simulink model "Milestone1"  (R2022b)
settings: Solver=VariableStepAuto  StartTime=0.0  StopTime=32  RelTol=1e-3
libraries: simulink x5
settings Model: Creator=nhatbuiminh  LastModifiedBy=nhatbuiminh

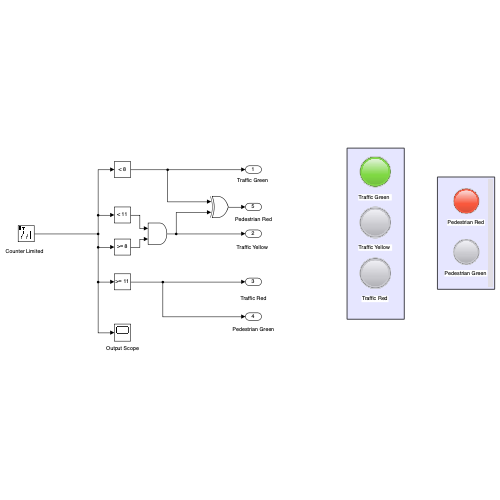
[thumbnail: Simulink's stored preview of the top-level diagram]
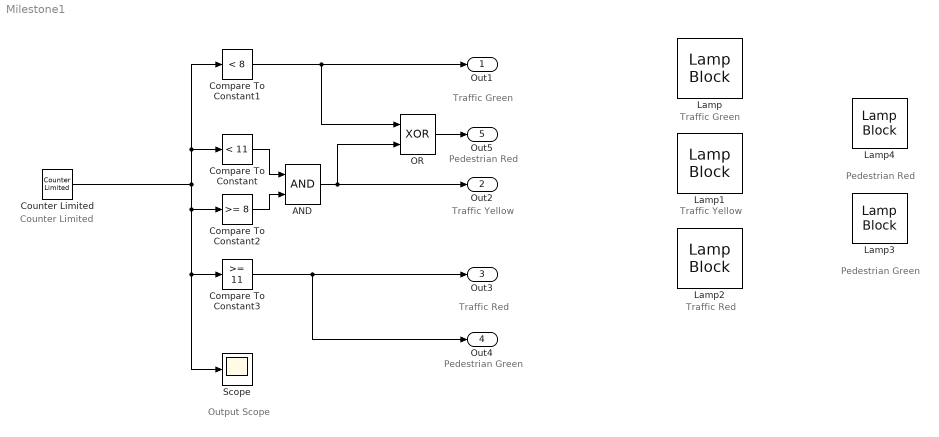
== system Milestone1 ==
  note: Pedestrian Green
  note: Traffic Red
  note: Traffic Yellow
  note: Traffic Green
  note: Traffic Green
  note: Traffic Yellow
  note: Traffic Red
  note: Pedestrian Green
  note: Pedestrian Red
  note: Pedestrian Red
  note: Output Scope
  note: Counter Limited
  AND : Logic  IconShape=distinctive  AllPortsSameDT=off  OutDataTypeStr=boolean
  Compare To Constant : simulink/Logic and Bit Operations/Compare To Constant  relop=<  const=11  OutDataTypeStr=boolean
  Compare To Constant1 : simulink/Logic and Bit Operations/Compare To Constant  relop=<  const=8  OutDataTypeStr=boolean
  Compare To Constant2 : simulink/Logic and Bit Operations/Compare To Constant  relop=>=  const=8  OutDataTypeStr=boolean
  Compare To Constant3 : simulink/Logic and Bit Operations/Compare To Constant  relop=>=  const=11  OutDataTypeStr=boolean
  Counter Limited : simulink/Sources/Counter Limited  uplimit=15  tsamp=1
  Lamp{,1..4} (5 alike) : LampBlock  LabelPosition=Hide
  OR : Logic  Operator=XOR  IconShape=distinctive  AllPortsSameDT=off  OutDataTypeStr=boolean
  Scope : Scope
  Out1 : Outport
  Out2 : Outport  Port=2
  Out3 : Outport  Port=3
  Out4 : Outport  Port=4
  Out5 : Outport  Port=5
  wires:
  Counter Limited/1 -> Compare To Constant1/1, Compare To Constant/1, Compare To Constant2/1, Compare To Constant3/1, Scope/1
  Compare To Constant2/1 -> AND/2
  Compare To Constant1/1 -> OR/1, Out1/1
  Compare To Constant/1 -> AND/1
  AND/1 -> OR/2, Out2/1
  Compare To Constant3/1 -> Out4/1, Out3/1
  OR/1 -> Out5/1
